simulink model "UAV_Research_Environment"  (R2025a)
settings: Solver=ode23t  StartTime=0.0  StopTime=130  MaxStep=2e-3  RelTol=1e-4  AbsTol=1e-3  EnableMultiTasking=on
InitFcn:
  | skipInitialization = false;
  | 
  | if evalin('base', ...
  |         'exist(''CONTROLLER_TUNING_ACTIVE'',''var'')')
  | 
  |     skipInitialization = evalin('base', ...
  |         'logical(CONTROLLER_TUNING_ACTIVE)');
  | end
  | 
  | if ~skipInitialization
  | 
  |     icraControllerPrepared = false;
  | 
  |     hasICRAVariables = evalin('base', ...
  |         ['exist(''AUTOPILOT'',''var'') && ' ...
  |          'exist(''ICRA_ACTIVE_CONTROLLER'',''var'') && ' ...
  |          'exist(''ICRA_ACTIVE_RUN_ID'',''var'')']);
  | 
  |     if hasICRAVariables
  | 
  |         icraControllerPrepared = evalin('base', ...
  |             ['isstruct(AUTOPILOT) && ' ...
  |              'isfield(AUTOPILOT,''info'') && ' ...
  |              'isfield(AUTOPILOT.info,''ICRAControllerID'') && ' ...
  |              'strcmp(string(AUTOPILOT.info.ICRAControllerID), ' ...
  |                     'string(ICRA_ACTIVE_CONTROLLER))']);
  | 
  |     end
  | 
  |     if icraControllerPrepared
  |         skipInitialization = true;
  |     end
  | end
  | 
  | if ~skipInitialization
  | 
  |     mdl = bdroot;
  | 
  |     mdl_file = get_param(mdl, 'FileName');
  | 
  |     project_root = fileparts(mdl_file);
  | 
  |     init_file = fullfile(project_root, 'initialize_project.m');
  | 
  |     if exist(init_file, 'file')
  | 
  |         run(init_file);
  | 
  |     else
  | 
  |         error('initialize_project.m was not found in the model folder.');
  | 
  |     end
  | end
values from neighbouring files (symbols this model uses):
  A_UAV = struct()    [UAV_analytical.m]
  AUTOPILOT = struct()    [UAV_autopilot.m]
  B_UAV = struct()    [UAV_block.m]
  D = A_UAV.source.propeller_diameter_m    [UAV_analytical.m]    (also in plot_controller_results.m = permute(                  D,                  order); plot_estimator_results.m = permute(              D,              order); plot_mission_results.m = permute(                  D,                  order); plot_touchdown_diagnostics.m = permute(                  D,                  order))
  OPERATOR_MODE = OPERATOR_MODE_MANUAL    [initialize_project.m]    (also in uav_remote_gui.m = uint8(0))
  P_ENV = struct()    [Environment.m]
  P_UAV = struct()    [UAV_simscape.m]
  s = sin(angle)    [uav_remote_gui.m]
  SENSOR = struct()    [UAV_sensors.m]
  TRAJECTORY_CONFIG = struct()    [UAV_trajectories.m]
  TRAJECTORY_ID = uint8(          trajectoryIDNumeric)    [UAV_trajectories.m]
  X = reshape(                  D,                  nt,                  [])    [plot_controller_results.m]    (also in plot_estimator_results.m = reshape(              D,              nt,              []); plot_mission_results.m; plot_touchdown_diagnostics.m; plot_trajectory_3d.m)
  Y = absolutePlanNED(1,:)    [plot_trajectory_3d.m]    (also in uav_remote_gui.m = positionNED(:,1))
  Z = landedCGDown -          absolutePlanNED(3,:)    [plot_trajectory_3d.m]    (also in uav_remote_gui.m = landedCGDown-positionNED(:,3))
undefined symbols (not defined in the file or in its folder): Acceleration_ref, F, fractalcoef, Light, MIL, Position_ref, Velocity_ref, Yaw_ref, YawRate_ref
libraries: sm_lib x49, nesl_utility x29, fl_lib x17, slpidlib x16, simulink x14, ee_lib x5, sdl_lib x4, aerolibwind2 x3, aerolibatmos2 x2, sensorbarometerlib x1, sensorgpslib x1, mspsensorlib x1
(part 6 of 9)

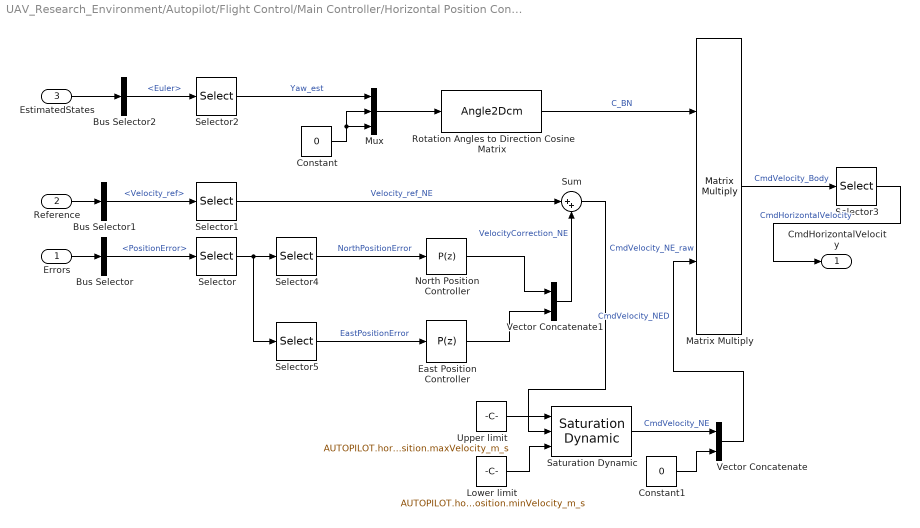
== system UAV_Research_Environment/Autopilot/Flight Control/Main Controller/Horizontal Position Control ==
  Errors : Inport
  Reference : Inport  Port=2
  EstimatedStates : Inport  Port=3
  Bus Selector : BusSelector  OutputSignals=PositionError
  Bus Selector1 : BusSelector  OutputSignals=Velocity_ref
  Bus Selector2 : BusSelector  OutputSignals=Attitude.Euler
  Constant : Constant  Value=0
  Constant1 : Constant  Value=0
  East Position Controller : slpidlib/PID Controller  Controller=P  Form=Parallel  TimeDomain=Discrete-time  UseExternalTs=off  SampleTime=AUTOPILOT.rate.controlSampleTime_s  IntegratorMethod=Forward Euler  FilterMethod=Forward Euler  ControllerParametersSource=internal  P=AUTOPILOT.horizontal.position.east.Kp  I=1  UseKiTs=off  D=0.550359987031017  UseExternalDerivativeSource=off  N=2.08014059923257  UseFilter=on  TunerSelectOption=Transfer Function Based (PID Tuner App)  InitialConditionSource=internal  InitialConditionForIntegrator=0  InitialConditionForFilter=0  DifferentiatorICPrevScaledInput=0  ExternalReset=level  TrackingMode=off  Kt=1  LimitOutput=off  SatLimitsSource=internal  UpperSaturationLimit=inf  LowerSaturationLimit=-inf  LinearizeAsGain=off  AntiWindupMode=none  Kb=1  LimitIntegrator=off  UpperIntegratorSaturationLimit=inf  LowerIntegratorSaturationLimit=-inf  POutMin=[]  POutMax=[]  IOutMin=[]  IOutMax=[]  DOutMin=[]  DOutMax=[]  NOutMin=[]  NOutMax=[]  SumOutMin=[]  SumOutMax=[]  SaturationOutMin=[]  SaturationOutMax=[]  PParamMin=[]  PParamMax=[]  IParamMin=[]  IParamMax=[]  DParamMin=[]  DParamMax=[]  NParamMin=[]  NParamMax=[]  KbParamMin=[]  KbParamMax=[]  KtParamMin=[]  KtParamMax=[]  KbOutMin=[]  KbOutMax=[]  KtOutMin=[]  KtOutMax=[]  IntegratorOutMin=[]  IntegratorOutMax=[]  FilterOutMin=[]  FilterOutMax=[]  SumI1OutMin=[]  SumI1OutMax=[]  SumI2OutMin=[]  SumI2OutMax=[]  SumI3OutMin=[]  SumI3OutMax=[]  SumI4OutMin=[]  SumI4OutMax=[]  SumDOutMin=[]  SumDOutMax=[]  DifferentiatorOutMin=[]  DifferentiatorOutMax=[]  FilterDiffOutCoefMin=[]  FilterDiffOutCoefMax=[]  ReciprocalOutMin=[]  ReciprocalOutMax=[]  SumDenOutMin=[]  SumDenOutMax=[]  SumNumOutMin=[]  SumNumOutMax=[]  DivideOutMin=[]  DivideOutMax=[]  UdiffTsProdOutMin=[]  UdiffTsProdOutMax=[]  NTsProdOutMin=[]  NTsProdOutMax=[]  UintegralTsProdOutMin=[]  UintegralTsProdOutMax=[]  UngainTsProdOutMin=[]  UngainTsProdOutMax=[]  ClampingZeroOutDataTypeStr=Inherit: Inherit via back propagation  ClampingZeroOutMin=[]  ClampingZeroOutMax=[]  FilterDenConstantOutDataTypeStr=Inherit: Inherit via back propagation  FilterDenConstantOutMin=[]  FilterDenConstantOutMax=[]  PCopyOutDataTypeStr=Inherit: Inherit via back propagation  PCopyOutMin=[]  PCopyOutMax=[]  NCopyOutDataTypeStr=Inherit: Inherit via back propagation  NCopyOutMin=[]  NCopyOutMax=[]  IntegratorContinuousStateAttributes=''  IntegratorStateMustResolveToSignalObject=off  IntegratorRTWStateStorageClass=Auto  FilterContinuousStateAttributes=''  FilterStateMustResolveToSignalObject=off  FilterRTWStateStorageClass=Auto  ParallelPVariant=InternalParameters  IdealPVariant=Disabled  IVariant=Disabled  DVariant=Disabled  IntegratorVariant=Disabled  SatVariant=Disabled  AWVariant=Disabled  PCopyVariant=Disabled  TRVariant=Disabled  FdbkBlocksVariant=Forward  IdealPFdbkVariant=Disabled  SatFdbkVariant=Disabled  DerivativeFilterVariant=Disabled  NVariant=Disabled  NCopyVariant=Disabled_SignalSpec  FilterICVariant=Disabled  IntegratorICVariant=Disabled  ExternalResetVariant=Disabled  TRSumVariant=Passthrough  SumFdbkVariant=Disabled  SumVariant=Passthrough_P  TsampFilterVariant=InternalTs  TsampNgainVariant=Passthrough  TsampIntegralVariant=Disabled_SignalSpec  ExternalSaturationOutDataTypeStr=Inherit: Same as second input  DerivativeSourceVariant=Disabled  PreIntVariant=InternalPreInt
      settings: LibrarySourceBlock=simulink/Discrete/Discrete PID Controller
  Lower limit : Constant  Value=AUTOPILOT.horizontal.position.minVelocity_m_s
  Matrix Multiply : Product  Multiplication=Matrix(*)
  Mux : Mux  Inputs=3
  North Position Controller : slpidlib/PID Controller  Controller=P  Form=Parallel  TimeDomain=Discrete-time  UseExternalTs=off  SampleTime=AUTOPILOT.rate.controlSampleTime_s  IntegratorMethod=Forward Euler  FilterMethod=Forward Euler  ControllerParametersSource=internal  P=AUTOPILOT.horizontal.position.north.Kp  I=1  UseKiTs=off  D=0  UseExternalDerivativeSource=off  N=100  UseFilter=on  TunerSelectOption=Transfer Function Based (PID Tuner App)  InitialConditionSource=internal  InitialConditionForIntegrator=0  InitialConditionForFilter=0  DifferentiatorICPrevScaledInput=0  ExternalReset=level  TrackingMode=off  Kt=1  LimitOutput=off  SatLimitsSource=internal  UpperSaturationLimit=inf  LowerSaturationLimit=-inf  LinearizeAsGain=off  AntiWindupMode=none  Kb=1  LimitIntegrator=off  UpperIntegratorSaturationLimit=inf  LowerIntegratorSaturationLimit=-inf  POutMin=[]  POutMax=[]  IOutMin=[]  IOutMax=[]  DOutMin=[]  DOutMax=[]  NOutMin=[]  NOutMax=[]  SumOutMin=[]  SumOutMax=[]  SaturationOutMin=[]  SaturationOutMax=[]  PParamMin=[]  PParamMax=[]  IParamMin=[]  IParamMax=[]  DParamMin=[]  DParamMax=[]  NParamMin=[]  NParamMax=[]  KbParamMin=[]  KbParamMax=[]  KtParamMin=[]  KtParamMax=[]  KbOutMin=[]  KbOutMax=[]  KtOutMin=[]  KtOutMax=[]  IntegratorOutMin=[]  IntegratorOutMax=[]  FilterOutMin=[]  FilterOutMax=[]  SumI1OutMin=[]  SumI1OutMax=[]  SumI2OutMin=[]  SumI2OutMax=[]  SumI3OutMin=[]  SumI3OutMax=[]  SumI4OutMin=[]  SumI4OutMax=[]  SumDOutMin=[]  SumDOutMax=[]  DifferentiatorOutMin=[]  DifferentiatorOutMax=[]  FilterDiffOutCoefMin=[]  FilterDiffOutCoefMax=[]  ReciprocalOutMin=[]  ReciprocalOutMax=[]  SumDenOutMin=[]  SumDenOutMax=[]  SumNumOutMin=[]  SumNumOutMax=[]  DivideOutMin=[]  DivideOutMax=[]  UdiffTsProdOutMin=[]  UdiffTsProdOutMax=[]  NTsProdOutMin=[]  NTsProdOutMax=[]  UintegralTsProdOutMin=[]  UintegralTsProdOutMax=[]  UngainTsProdOutMin=[]  UngainTsProdOutMax=[]  ClampingZeroOutDataTypeStr=Inherit: Inherit via back propagation  ClampingZeroOutMin=[]  ClampingZeroOutMax=[]  FilterDenConstantOutDataTypeStr=Inherit: Inherit via back propagation  FilterDenConstantOutMin=[]  FilterDenConstantOutMax=[]  PCopyOutDataTypeStr=Inherit: Inherit via back propagation  PCopyOutMin=[]  PCopyOutMax=[]  NCopyOutDataTypeStr=Inherit: Inherit via back propagation  NCopyOutMin=[]  NCopyOutMax=[]  IntegratorContinuousStateAttributes=''  IntegratorStateMustResolveToSignalObject=off  IntegratorRTWStateStorageClass=Auto  FilterContinuousStateAttributes=''  FilterStateMustResolveToSignalObject=off  FilterRTWStateStorageClass=Auto  ParallelPVariant=InternalParameters  IdealPVariant=Disabled  IVariant=Disabled  DVariant=Disabled  IntegratorVariant=Disabled  SatVariant=Disabled  AWVariant=Disabled  PCopyVariant=Disabled  TRVariant=Disabled  FdbkBlocksVariant=Forward  IdealPFdbkVariant=Disabled  SatFdbkVariant=Disabled  DerivativeFilterVariant=Disabled  NVariant=Disabled  NCopyVariant=Disabled_SignalSpec  FilterICVariant=Disabled  IntegratorICVariant=Disabled  ExternalResetVariant=Disabled  TRSumVariant=Passthrough  SumFdbkVariant=Disabled  SumVariant=Passthrough_P  TsampFilterVariant=InternalTs  TsampNgainVariant=Passthrough  TsampIntegralVariant=Disabled_SignalSpec  ExternalSaturationOutDataTypeStr=Inherit: Same as second input  DerivativeSourceVariant=Disabled  PreIntVariant=InternalPreInt
      settings: LibrarySourceBlock=simulink/Discrete/Discrete PID Controller
  Rotation Angles to Direction Cosine Matrix : Angle2Dcm
      settings: AttributesFormatString=Rotation Order: %<rotationOrder>
  Saturation Dynamic : simulink/Discontinuities/Saturation Dynamic  OutMin=[]  OutMax=[]  OutDataTypeStr=Inherit: Same as second input  OutDataType=fixdt(1, 16)  OutScaling=2^-10  DoSatur=off
  Selector : Selector  InputPortWidth=3  IndexOptions=Index vector (dialog)  Indices=[1 2]  OutputSizes=1
  Selector1 : Selector  InputPortWidth=3  IndexOptions=Index vector (dialog)  Indices=[1 2]  OutputSizes=1
  Selector2 : Selector  InputPortWidth=3  IndexOptions=Index vector (dialog)  Indices=3  OutputSizes=1
  Selector3 : Selector  InputPortWidth=3  IndexOptions=Index vector (dialog)  Indices=[1 2]  OutputSizes=1
  Selector4 : Selector  InputPortWidth=2  IndexOptions=Index vector (dialog)  Indices=1  OutputSizes=1
  Selector5 : Selector  InputPortWidth=2  IndexOptions=Index vector (dialog)  Indices=2  OutputSizes=1
  Sum : Sum  Inputs=|++
  Upper limit : Constant  Value=AUTOPILOT.horizontal.position.maxVelocity_m_s
  Vector Concatenate : Concatenate
  Vector Concatenate1 : Concatenate
  CmdHorizontalVelocity : Outport
  wires:
  Errors/1 -> Bus Selector/1
  Bus Selector/1 -> Selector/1  "<PositionError>"
  Reference/1 -> Bus Selector1/1
  Bus Selector1/1 -> Selector1/1  "<Velocity_ref>"
  EstimatedStates/1 -> Bus Selector2/1
  Bus Selector2/1 -> Selector2/1  "<Euler>"
  Selector/1 -> Selector5/1, Selector4/1
  Vector Concatenate1/1 -> Sum/2  "VelocityCorrection_NE"
  Selector1/1 -> Sum/1  "Velocity_ref_NE"
  Sum/1 -> Saturation Dynamic/2  "CmdVelocity_NE_raw"
  Saturation Dynamic/1 -> Vector Concatenate/1  "CmdVelocity_NE"
  Upper limit/1 -> Saturation Dynamic/1
  Lower limit/1 -> Saturation Dynamic/3
  Selector2/1 -> Mux/1  "Yaw_est"
  Constant/1 -> Mux/2, Mux/3
  Mux/1 -> Rotation Angles to Direction Cosine Matrix/1
  Rotation Angles to Direction Cosine Matrix/1 -> Matrix Multiply/1  "C_BN"
  Constant1/1 -> Vector Concatenate/2
  Vector Concatenate/1 -> Matrix Multiply/2  "CmdVelocity_NED"
  Matrix Multiply/1 -> Selector3/1  "CmdVelocity_Body"
  Selector3/1 -> CmdHorizontalVelocity/1  "CmdHorizontalVelocity"
  Selector4/1 -> North Position Controller/1  "NorthPositionError"
  Selector5/1 -> East Position Controller/1  "EastPositionError"
  North Position Controller/1 -> Vector Concatenate1/1
  East Position Controller/1 -> Vector Concatenate1/2

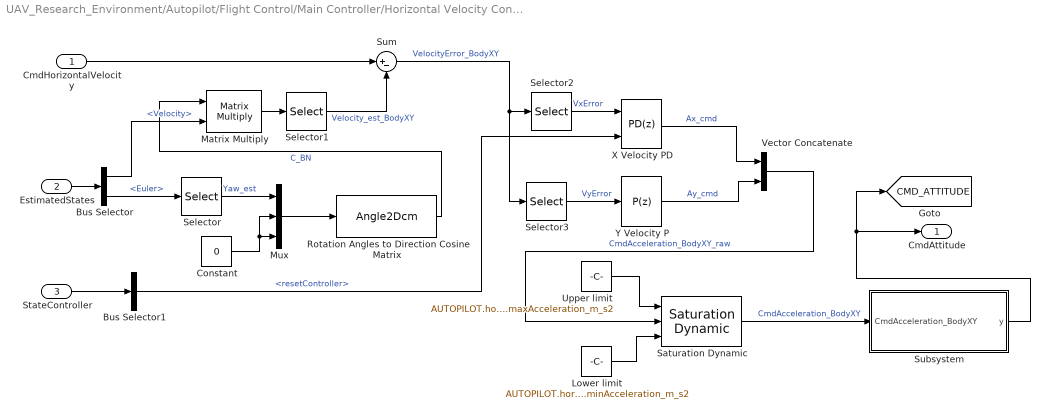
== system UAV_Research_Environment/Autopilot/Flight Control/Main Controller/Horizontal Velocity Control ==
  CmdHorizontalVelocity : Inport
  EstimatedStates : Inport  Port=2
  StateController : Inport  Port=3
  Bus Selector : BusSelector  OutputSignals=Velocity,Attitude.Euler
  Bus Selector1 : BusSelector  OutputSignals=resetController
  Constant : Constant  Value=0
  Lower limit : Constant  Value=AUTOPILOT.horizontal.velocity.minAcceleration_m_s2
  Matrix Multiply : Product  Multiplication=Matrix(*)
  Mux : Mux  Inputs=3
  Rotation Angles to Direction Cosine Matrix : Angle2Dcm
      settings: AttributesFormatString=Rotation Order: %<rotationOrder>
  Saturation Dynamic : simulink/Discontinuities/Saturation Dynamic  OutMin=[]  OutMax=[]  OutDataTypeStr=Inherit: Same as second input  OutDataType=fixdt(1, 16)  OutScaling=2^-10  DoSatur=off
  Selector : Selector  InputPortWidth=3  IndexOptions=Index vector (dialog)  Indices=3  OutputSizes=1
  Selector1 : Selector  InputPortWidth=3  IndexOptions=Index vector (dialog)  Indices=[1 2]  OutputSizes=1
  Selector2 : Selector  InputPortWidth=2  IndexOptions=Index vector (dialog)  Indices=1  OutputSizes=1
  Selector3 : Selector  InputPortWidth=2  IndexOptions=Index vector (dialog)  Indices=2  OutputSizes=1
  Subsystem : Subsystem
  Sum : Sum  Inputs=|+-
  Upper limit : Constant  Value=AUTOPILOT.horizontal.velocity.maxAcceleration_m_s2
  Vector Concatenate : Concatenate
  X Velocity PD : slpidlib/PID Controller  Controller=PD  Form=Parallel  TimeDomain=Discrete-time  UseExternalTs=off  SampleTime=AUTOPILOT.rate.controlSampleTime_s  IntegratorMethod=Forward Euler  FilterMethod=Forward Euler  ControllerParametersSource=internal  P=AUTOPILOT.horizontal.velocity.x.Kp  I=AUTOPILOT.horizontal.velocity.Ki  UseKiTs=off  D=AUTOPILOT.horizontal.velocity.x.Kd  UseExternalDerivativeSource=off  N=AUTOPILOT.horizontal.velocity.x.N  UseFilter=on  TunerSelectOption=Transfer Function Based (PID Tuner App)  InitialConditionSource=internal  InitialConditionForIntegrator=0  InitialConditionForFilter=0  DifferentiatorICPrevScaledInput=0  ExternalReset=level  TrackingMode=off  Kt=1  LimitOutput=off  SatLimitsSource=internal  UpperSaturationLimit=inf  LowerSaturationLimit=-inf  LinearizeAsGain=off  AntiWindupMode=none  Kb=1  LimitIntegrator=off  UpperIntegratorSaturationLimit=inf  LowerIntegratorSaturationLimit=-inf  POutMin=[]  POutMax=[]  IOutMin=[]  IOutMax=[]  DOutMin=[]  DOutMax=[]  NOutMin=[]  NOutMax=[]  SumOutMin=[]  SumOutMax=[]  SaturationOutMin=[]  SaturationOutMax=[]  PParamMin=[]  PParamMax=[]  IParamMin=[]  IParamMax=[]  DParamMin=[]  DParamMax=[]  NParamMin=[]  NParamMax=[]  KbParamMin=[]  KbParamMax=[]  KtParamMin=[]  KtParamMax=[]  KbOutMin=[]  KbOutMax=[]  KtOutMin=[]  KtOutMax=[]  IntegratorOutMin=[]  IntegratorOutMax=[]  FilterOutMin=[]  FilterOutMax=[]  SumI1OutMin=[]  SumI1OutMax=[]  SumI2OutMin=[]  SumI2OutMax=[]  SumI3OutMin=[]  SumI3OutMax=[]  SumI4OutMin=[]  SumI4OutMax=[]  SumDOutMin=[]  SumDOutMax=[]  DifferentiatorOutMin=[]  DifferentiatorOutMax=[]  FilterDiffOutCoefMin=[]  FilterDiffOutCoefMax=[]  ReciprocalOutMin=[]  ReciprocalOutMax=[]  SumDenOutMin=[]  SumDenOutMax=[]  SumNumOutMin=[]  SumNumOutMax=[]  DivideOutMin=[]  DivideOutMax=[]  UdiffTsProdOutMin=[]  UdiffTsProdOutMax=[]  NTsProdOutMin=[]  NTsProdOutMax=[]  UintegralTsProdOutMin=[]  UintegralTsProdOutMax=[]  UngainTsProdOutMin=[]  UngainTsProdOutMax=[]  ClampingZeroOutDataTypeStr=Inherit: Inherit via back propagation  ClampingZeroOutMin=[]  ClampingZeroOutMax=[]  FilterDenConstantOutDataTypeStr=Inherit: Inherit via back propagation  FilterDenConstantOutMin=[]  FilterDenConstantOutMax=[]  PCopyOutDataTypeStr=Inherit: Inherit via back propagation  PCopyOutMin=[]  PCopyOutMax=[]  NCopyOutDataTypeStr=Inherit: Inherit via back propagation  NCopyOutMin=[]  NCopyOutMax=[]  IntegratorContinuousStateAttributes=''  IntegratorStateMustResolveToSignalObject=off  IntegratorRTWStateStorageClass=Auto  FilterContinuousStateAttributes=''  FilterStateMustResolveToSignalObject=off  FilterRTWStateStorageClass=Auto  ParallelPVariant=InternalParameters  IdealPVariant=Disabled  IVariant=Disabled  DVariant=InternalParameters  IntegratorVariant=Disabled  SatVariant=Disabled  AWVariant=Disabled  PCopyVariant=Disabled  TRVariant=Disabled  FdbkBlocksVariant=Forward  IdealPFdbkVariant=Disabled  SatFdbkVariant=Disabled  DerivativeFilterVariant=ForwardEulerFilter  NVariant=InternalParameters  NCopyVariant=Disabled  FilterICVariant=InternalICsFilter  IntegratorICVariant=Disabled  ExternalResetVariant=ExternalReset  TRSumVariant=Passthrough  SumFdbkVariant=Disabled  SumVariant=Sum_PD  TsampFilterVariant=InternalTs  TsampNgainVariant=Passthrough  TsampIntegralVariant=Disabled_SignalSpec  ExternalSaturationOutDataTypeStr=Inherit: Same as second input  DerivativeSourceVariant=ErrorSignal  PreIntVariant=InternalPreInt
      settings: LibrarySourceBlock=simulink/Discrete/Discrete PID Controller
  Y Velocity P : slpidlib/PID Controller  Controller=P  Form=Parallel  TimeDomain=Discrete-time  UseExternalTs=off  SampleTime=AUTOPILOT.rate.controlSampleTime_s  IntegratorMethod=Forward Euler  FilterMethod=Forward Euler  ControllerParametersSource=internal  P=AUTOPILOT.horizontal.velocity.y.Kp  I=AUTOPILOT.horizontal.velocity.Ki  UseKiTs=off  D=AUTOPILOT.horizontal.velocity.Kd  UseExternalDerivativeSource=off  N=AUTOPILOT.horizontal.velocity.N  UseFilter=on  TunerSelectOption=Transfer Function Based (PID Tuner App)  InitialConditionSource=internal  InitialConditionForIntegrator=0  InitialConditionForFilter=0  DifferentiatorICPrevScaledInput=0  ExternalReset=level  TrackingMode=off  Kt=1  LimitOutput=off  SatLimitsSource=internal  UpperSaturationLimit=inf  LowerSaturationLimit=-inf  LinearizeAsGain=off  AntiWindupMode=none  Kb=1  LimitIntegrator=off  UpperIntegratorSaturationLimit=inf  LowerIntegratorSaturationLimit=-inf  POutMin=[]  POutMax=[]  IOutMin=[]  IOutMax=[]  DOutMin=[]  DOutMax=[]  NOutMin=[]  NOutMax=[]  SumOutMin=[]  SumOutMax=[]  SaturationOutMin=[]  SaturationOutMax=[]  PParamMin=[]  PParamMax=[]  IParamMin=[]  IParamMax=[]  DParamMin=[]  DParamMax=[]  NParamMin=[]  NParamMax=[]  KbParamMin=[]  KbParamMax=[]  KtParamMin=[]  KtParamMax=[]  KbOutMin=[]  KbOutMax=[]  KtOutMin=[]  KtOutMax=[]  IntegratorOutMin=[]  IntegratorOutMax=[]  FilterOutMin=[]  FilterOutMax=[]  SumI1OutMin=[]  SumI1OutMax=[]  SumI2OutMin=[]  SumI2OutMax=[]  SumI3OutMin=[]  SumI3OutMax=[]  SumI4OutMin=[]  SumI4OutMax=[]  SumDOutMin=[]  SumDOutMax=[]  DifferentiatorOutMin=[]  DifferentiatorOutMax=[]  FilterDiffOutCoefMin=[]  FilterDiffOutCoefMax=[]  ReciprocalOutMin=[]  ReciprocalOutMax=[]  SumDenOutMin=[]  SumDenOutMax=[]  SumNumOutMin=[]  SumNumOutMax=[]  DivideOutMin=[]  DivideOutMax=[]  UdiffTsProdOutMin=[]  UdiffTsProdOutMax=[]  NTsProdOutMin=[]  NTsProdOutMax=[]  UintegralTsProdOutMin=[]  UintegralTsProdOutMax=[]  UngainTsProdOutMin=[]  UngainTsProdOutMax=[]  ClampingZeroOutDataTypeStr=Inherit: Inherit via back propagation  ClampingZeroOutMin=[]  ClampingZeroOutMax=[]  FilterDenConstantOutDataTypeStr=Inherit: Inherit via back propagation  FilterDenConstantOutMin=[]  FilterDenConstantOutMax=[]  PCopyOutDataTypeStr=Inherit: Inherit via back propagation  PCopyOutMin=[]  PCopyOutMax=[]  NCopyOutDataTypeStr=Inherit: Inherit via back propagation  NCopyOutMin=[]  NCopyOutMax=[]  IntegratorContinuousStateAttributes=''  IntegratorStateMustResolveToSignalObject=off  IntegratorRTWStateStorageClass=Auto  FilterContinuousStateAttributes=''  FilterStateMustResolveToSignalObject=off  FilterRTWStateStorageClass=Auto  ParallelPVariant=InternalParameters  IdealPVariant=Disabled  IVariant=Disabled  DVariant=Disabled  IntegratorVariant=Disabled  SatVariant=Disabled  AWVariant=Disabled  PCopyVariant=Disabled  TRVariant=Disabled  FdbkBlocksVariant=Forward  IdealPFdbkVariant=Disabled  SatFdbkVariant=Disabled  DerivativeFilterVariant=Disabled  NVariant=Disabled  NCopyVariant=Disabled_SignalSpec  FilterICVariant=Disabled  IntegratorICVariant=Disabled  ExternalResetVariant=Disabled  TRSumVariant=Passthrough  SumFdbkVariant=Disabled  SumVariant=Passthrough_P  TsampFilterVariant=InternalTs  TsampNgainVariant=Passthrough  TsampIntegralVariant=Disabled_SignalSpec  ExternalSaturationOutDataTypeStr=Inherit: Same as second input  DerivativeSourceVariant=Disabled  PreIntVariant=InternalPreInt
      settings: LibrarySourceBlock=simulink/Discrete/Discrete PID Controller
  CmdAttitude : Outport
  tag scope: CMD_ATTITUDE=global
  wires:
  EstimatedStates/1 -> Bus Selector/1
  StateController/1 -> Bus Selector1/1
  Bus Selector/2 -> Selector/1  "<Euler>"
  Selector/1 -> Mux/1  "Yaw_est"
  Constant/1 -> Mux/2, Mux/3
  Mux/1 -> Rotation Angles to Direction Cosine Matrix/1
  Rotation Angles to Direction Cosine Matrix/1 -> Matrix Multiply/1  "C_BN"
  Bus Selector/1 -> Matrix Multiply/2  "<Velocity>"
  Matrix Multiply/1 -> Selector1/1
  Selector1/1 -> Sum/2  "Velocity_est_BodyXY"
  CmdHorizontalVelocity/1 -> Sum/1
  Sum/1 -> Selector3/1, Selector2/1  "VelocityError_BodyXY"
  Bus Selector1/1 -> X Velocity PD/2  "<resetController>"
  Vector Concatenate/1 -> Saturation Dynamic/2  "CmdAcceleration_BodyXY_raw"
  Upper limit/1 -> Saturation Dynamic/1
  Lower limit/1 -> Saturation Dynamic/3
  Saturation Dynamic/1 -> Subsystem/1(CmdAcceleration_BodyXY)  "CmdAcceleration_BodyXY"
  Selector2/1 -> X Velocity PD/1  "VxError"
  Selector3/1 -> Y Velocity P/1  "VyError"
  Y Velocity P/1 -> Vector Concatenate/2  "Ay_cmd"
  Subsystem/1(y) -> [CMD_ATTITUDE], CmdAttitude/1
  X Velocity PD/1 -> Vector Concatenate/1  "Ax_cmd"

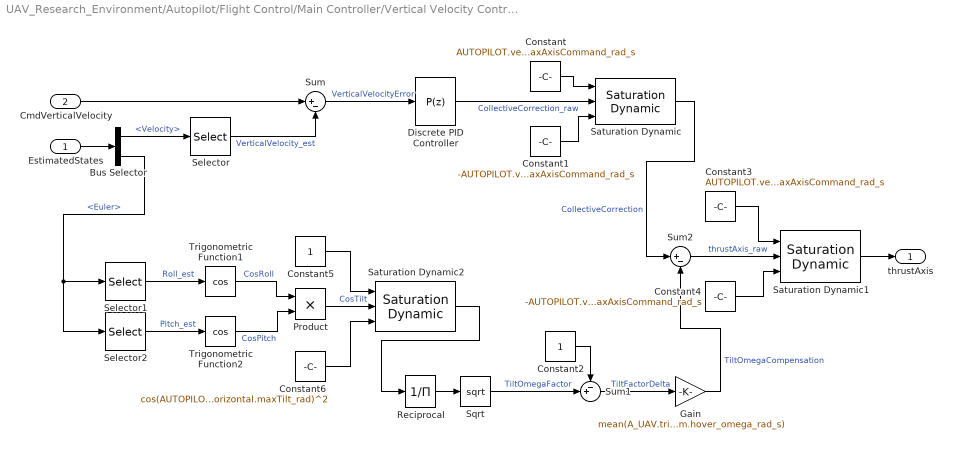
== system UAV_Research_Environment/Autopilot/Flight Control/Main Controller/Vertical Velocity Control ==
  EstimatedStates : Inport
  CmdVerticalVelocity : Inport  Port=2
  Bus Selector : BusSelector  OutputSignals=Velocity,Attitude.Euler
  Constant : Constant  Value=AUTOPILOT.vertical.velocity.maxAxisCommand_rad_s
  Constant1 : Constant  Value=-AUTOPILOT.vertical.velocity.maxAxisCommand_rad_s
  Constant2 : Constant
  Constant3 : Constant  Value=AUTOPILOT.vertical.velocity.maxAxisCommand_rad_s
  Constant4 : Constant  Value=-AUTOPILOT.vertical.velocity.maxAxisCommand_rad_s
  Constant5 : Constant
  Constant6 : Constant  Value=cos(AUTOPILOT.horizontal.maxTilt_rad)^2
  Discrete PID Controller : slpidlib/PID Controller  Controller=P  Form=Parallel  TimeDomain=Discrete-time  UseExternalTs=off  SampleTime=AUTOPILOT.rate.controlSampleTime_s  IntegratorMethod=Forward Euler  FilterMethod=Forward Euler  ControllerParametersSource=internal  P=AUTOPILOT.vertical.velocity.Kp  I=AUTOPILOT.vertical.velocity.Ki  UseKiTs=off  D=AUTOPILOT.vertical.velocity.Kd  UseExternalDerivativeSource=off  N=AUTOPILOT.vertical.velocity.N  UseFilter=on  TunerSelectOption=Transfer Function Based (PID Tuner App)  InitialConditionSource=internal  InitialConditionForIntegrator=0  InitialConditionForFilter=0  DifferentiatorICPrevScaledInput=0  ExternalReset=level  TrackingMode=off  Kt=1  LimitOutput=off  SatLimitsSource=internal  UpperSaturationLimit=inf  LowerSaturationLimit=-inf  LinearizeAsGain=off  AntiWindupMode=clamping  Kb=1  LimitIntegrator=on  UpperIntegratorSaturationLimit=AUTOPILOT.vertical.velocity.integratorUpperLimit  LowerIntegratorSaturationLimit=AUTOPILOT.vertical.velocity.integratorLowerLimit  POutMin=[]  POutMax=[]  IOutMin=[]  IOutMax=[]  DOutMin=[]  DOutMax=[]  NOutMin=[]  NOutMax=[]  SumOutMin=[]  SumOutMax=[]  SaturationOutMin=[]  SaturationOutMax=[]  PParamMin=[]  PParamMax=[]  IParamMin=[]  IParamMax=[]  DParamMin=[]  DParamMax=[]  NParamMin=[]  NParamMax=[]  KbParamMin=[]  KbParamMax=[]  KtParamMin=[]  KtParamMax=[]  KbOutMin=[]  KbOutMax=[]  KtOutMin=[]  KtOutMax=[]  IntegratorOutMin=[]  IntegratorOutMax=[]  FilterOutMin=[]  FilterOutMax=[]  SumI1OutMin=[]  SumI1OutMax=[]  SumI2OutMin=[]  SumI2OutMax=[]  SumI3OutMin=[]  SumI3OutMax=[]  SumI4OutMin=[]  SumI4OutMax=[]  SumDOutMin=[]  SumDOutMax=[]  DifferentiatorOutMin=[]  DifferentiatorOutMax=[]  FilterDiffOutCoefMin=[]  FilterDiffOutCoefMax=[]  ReciprocalOutMin=[]  ReciprocalOutMax=[]  SumDenOutMin=[]  SumDenOutMax=[]  SumNumOutMin=[]  SumNumOutMax=[]  DivideOutMin=[]  DivideOutMax=[]  UdiffTsProdOutMin=[]  UdiffTsProdOutMax=[]  NTsProdOutMin=[]  NTsProdOutMax=[]  UintegralTsProdOutMin=[]  UintegralTsProdOutMax=[]  UngainTsProdOutMin=[]  UngainTsProdOutMax=[]  ClampingZeroOutDataTypeStr=Inherit: Inherit via back propagation  ClampingZeroOutMin=[]  ClampingZeroOutMax=[]  FilterDenConstantOutDataTypeStr=Inherit: Inherit via back propagation  FilterDenConstantOutMin=[]  FilterDenConstantOutMax=[]  PCopyOutDataTypeStr=Inherit: Inherit via back propagation  PCopyOutMin=[]  PCopyOutMax=[]  NCopyOutDataTypeStr=Inherit: Inherit via back propagation  NCopyOutMin=[]  NCopyOutMax=[]  IntegratorContinuousStateAttributes=''  IntegratorStateMustResolveToSignalObject=off  IntegratorRTWStateStorageClass=Auto  FilterContinuousStateAttributes=''  FilterStateMustResolveToSignalObject=off  FilterRTWStateStorageClass=Auto  ParallelPVariant=InternalParameters  IdealPVariant=Disabled  IVariant=Disabled  DVariant=Disabled  IntegratorVariant=Disabled  SatVariant=Disabled  AWVariant=Disabled  PCopyVariant=Disabled  TRVariant=Disabled  FdbkBlocksVariant=Forward  IdealPFdbkVariant=Disabled  SatFdbkVariant=Disabled  DerivativeFilterVariant=Disabled  NVariant=Disabled  NCopyVariant=Disabled_SignalSpec  FilterICVariant=Disabled  IntegratorICVariant=Disabled  ExternalResetVariant=Disabled  TRSumVariant=Passthrough  SumFdbkVariant=Disabled  SumVariant=Passthrough_P  TsampFilterVariant=InternalTs  TsampNgainVariant=Passthrough  TsampIntegralVariant=Disabled_SignalSpec  ExternalSaturationOutDataTypeStr=Inherit: Same as second input  DerivativeSourceVariant=Disabled  PreIntVariant=InternalPreInt
      settings: LibrarySourceBlock=simulink/Discrete/Discrete PID Controller
  Gain : Gain  Gain=mean(A_UAV.trim.hover_omega_rad_s)
  Product : Product
  Reciprocal : Product  Inputs=/
  Saturation Dynamic : simulink/Discontinuities/Saturation Dynamic  OutMin=[]  OutMax=[]  OutDataTypeStr=Inherit: Same as second input  OutDataType=fixdt(1, 16)  OutScaling=2^-10  DoSatur=off
  Saturation Dynamic1 : simulink/Discontinuities/Saturation Dynamic  OutMin=[]  OutMax=[]  OutDataTypeStr=Inherit: Same as second input  OutDataType=fixdt(1, 16)  OutScaling=2^-10  DoSatur=off
  Saturation Dynamic2 : simulink/Discontinuities/Saturation Dynamic  OutMin=[]  OutMax=[]  OutDataTypeStr=Inherit: Same as second input  OutDataType=fixdt(1, 16)  OutScaling=2^-10  DoSatur=off
  Selector : Selector  InputPortWidth=3  IndexOptions=Index vector (dialog)  Indices=3  OutputSizes=1
  Selector1 : Selector  InputPortWidth=3  IndexOptions=Index vector (dialog)  Indices=1  OutputSizes=1
  Selector2 : Selector  InputPortWidth=3  IndexOptions=Index vector (dialog)  Indices=2  OutputSizes=1
  Sqrt : Sqrt
  Sum : Sum  Inputs=|+-
  Sum1 : Sum  Inputs=-+|
  Sum2 : Sum  Inputs=|+-
  Trigonometric Function1 : Trigonometry  Operator=cos
  Trigonometric Function2 : Trigonometry  Operator=cos
  thrustAxis : Outport
  wires:
  EstimatedStates/1 -> Bus Selector/1
  Bus Selector/1 -> Selector/1  "<Velocity>"
  Selector/1 -> Sum/2  "VerticalVelocity_est"
  CmdVerticalVelocity/1 -> Sum/1
  Sum/1 -> Discrete PID Controller/1  "VerticalVelocityError"
  Discrete PID Controller/1 -> Saturation Dynamic/2  "CollectiveCorrection_raw"
  Constant/1 -> Saturation Dynamic/1
  Constant1/1 -> Saturation Dynamic/3
  Saturation Dynamic/1 -> Sum2/1  "CollectiveCorrection"
  Selector1/1 -> Trigonometric Function1/1  "Roll_est"
  Selector2/1 -> Trigonometric Function2/1  "Pitch_est"
  Trigonometric Function1/1 -> Product/1  "CosRoll"
  Trigonometric Function2/1 -> Product/2  "CosPitch"
  Reciprocal/1 -> Sqrt/1
  Bus Selector/2 -> Selector2/1, Selector1/1  "<Euler>"
  Sum1/1 -> Gain/1  "TiltFactorDelta"
  Gain/1 -> Sum2/2  "TiltOmegaCompensation"
  Sum2/1 -> Saturation Dynamic1/2  "thrustAxis_raw"
  Saturation Dynamic1/1 -> thrustAxis/1
  Constant3/1 -> Saturation Dynamic1/1
  Constant4/1 -> Saturation Dynamic1/3
  Product/1 -> Saturation Dynamic2/2  "CosTilt"
  Saturation Dynamic2/1 -> Reciprocal/1
  Constant5/1 -> Saturation Dynamic2/1
  Constant6/1 -> Saturation Dynamic2/3
  Sqrt/1 -> Sum1/2  "TiltOmegaFactor"
  Constant2/1 -> Sum1/1

== system UAV_Research_Environment/Autopilot/Flight Control/Main Controller/Yaw Angle Control ==
  Errors : Inport
  Reference : Inport  Port=2
  Bus Selector : BusSelector  OutputSignals=YawError
  Bus Selector1 : BusSelector  OutputSignals=YawRate_ref
  Constant : Constant  Value=AUTOPILOT.yaw.angle.maxYawRate_rad_s
  Constant1 : Constant  Value=AUTOPILOT.yaw.angle.minYawRate_rad_s
  Discrete PID Controller : slpidlib/PID Controller  Controller=P  Form=Parallel  TimeDomain=Discrete-time  UseExternalTs=off  SampleTime=AUTOPILOT.rate.controlSampleTime_s  IntegratorMethod=Forward Euler  FilterMethod=Forward Euler  ControllerParametersSource=internal  P=AUTOPILOT.yaw.angle.Kp  I=AUTOPILOT.yaw.angle.Ki  UseKiTs=off  D=AUTOPILOT.yaw.angle.Kd  UseExternalDerivativeSource=off  N=AUTOPILOT.yaw.angle.N  UseFilter=on  TunerSelectOption=Transfer Function Based (PID Tuner App)  InitialConditionSource=internal  InitialConditionForIntegrator=0  InitialConditionForFilter=0  DifferentiatorICPrevScaledInput=0  ExternalReset=level  TrackingMode=off  Kt=1  LimitOutput=off  SatLimitsSource=internal  UpperSaturationLimit=inf  LowerSaturationLimit=-inf  LinearizeAsGain=off  AntiWindupMode=none  Kb=1  LimitIntegrator=off  UpperIntegratorSaturationLimit=inf  LowerIntegratorSaturationLimit=-inf  POutMin=[]  POutMax=[]  IOutMin=[]  IOutMax=[]  DOutMin=[]  DOutMax=[]  NOutMin=[]  NOutMax=[]  SumOutMin=[]  SumOutMax=[]  SaturationOutMin=[]  SaturationOutMax=[]  PParamMin=[]  PParamMax=[]  IParamMin=[]  IParamMax=[]  DParamMin=[]  DParamMax=[]  NParamMin=[]  NParamMax=[]  KbParamMin=[]  KbParamMax=[]  KtParamMin=[]  KtParamMax=[]  KbOutMin=[]  KbOutMax=[]  KtOutMin=[]  KtOutMax=[]  IntegratorOutMin=[]  IntegratorOutMax=[]  FilterOutMin=[]  FilterOutMax=[]  SumI1OutMin=[]  SumI1OutMax=[]  SumI2OutMin=[]  SumI2OutMax=[]  SumI3OutMin=[]  SumI3OutMax=[]  SumI4OutMin=[]  SumI4OutMax=[]  SumDOutMin=[]  SumDOutMax=[]  DifferentiatorOutMin=[]  DifferentiatorOutMax=[]  FilterDiffOutCoefMin=[]  FilterDiffOutCoefMax=[]  ReciprocalOutMin=[]  ReciprocalOutMax=[]  SumDenOutMin=[]  SumDenOutMax=[]  SumNumOutMin=[]  SumNumOutMax=[]  DivideOutMin=[]  DivideOutMax=[]  UdiffTsProdOutMin=[]  UdiffTsProdOutMax=[]  NTsProdOutMin=[]  NTsProdOutMax=[]  UintegralTsProdOutMin=[]  UintegralTsProdOutMax=[]  UngainTsProdOutMin=[]  UngainTsProdOutMax=[]  ClampingZeroOutDataTypeStr=Inherit: Inherit via back propagation  ClampingZeroOutMin=[]  ClampingZeroOutMax=[]  FilterDenConstantOutDataTypeStr=Inherit: Inherit via back propagation  FilterDenConstantOutMin=[]  FilterDenConstantOutMax=[]  PCopyOutDataTypeStr=Inherit: Inherit via back propagation  PCopyOutMin=[]  PCopyOutMax=[]  NCopyOutDataTypeStr=Inherit: Inherit via back propagation  NCopyOutMin=[]  NCopyOutMax=[]  IntegratorContinuousStateAttributes=''  IntegratorStateMustResolveToSignalObject=off  IntegratorRTWStateStorageClass=Auto  FilterContinuousStateAttributes=''  FilterStateMustResolveToSignalObject=off  FilterRTWStateStorageClass=Auto  ParallelPVariant=InternalParameters  IdealPVariant=Disabled  IVariant=Disabled  DVariant=Disabled  IntegratorVariant=Disabled  SatVariant=Disabled  AWVariant=Disabled  PCopyVariant=Disabled  TRVariant=Disabled  FdbkBlocksVariant=Forward  IdealPFdbkVariant=Disabled  SatFdbkVariant=Disabled  DerivativeFilterVariant=Disabled  NVariant=Disabled  NCopyVariant=Disabled_SignalSpec  FilterICVariant=Disabled  IntegratorICVariant=Disabled  ExternalResetVariant=Disabled  TRSumVariant=Passthrough  SumFdbkVariant=Disabled  SumVariant=Passthrough_P  TsampFilterVariant=InternalTs  TsampNgainVariant=Passthrough  TsampIntegralVariant=Disabled_SignalSpec  ExternalSaturationOutDataTypeStr=Inherit: Same as second input  DerivativeSourceVariant=Disabled  PreIntVariant=InternalPreInt
      settings: LibrarySourceBlock=simulink/Discrete/Discrete PID Controller
  Saturation Dynamic : simulink/Discontinuities/Saturation Dynamic  OutMin=[]  OutMax=[]  OutDataTypeStr=Inherit: Same as second input  OutDataType=fixdt(1, 16)  OutScaling=2^-10  DoSatur=off
  Sum : Sum  Inputs=|++
  CmdYawAngleRate : Outport
  wires:
  Errors/1 -> Bus Selector/1
  Reference/1 -> Bus Selector1/1
  Discrete PID Controller/1 -> Sum/1  "YawRateCorrection"
  Bus Selector/1 -> Discrete PID Controller/1  "<YawError>"
  Bus Selector1/1 -> Sum/2  "<YawRate_ref>"
  Sum/1 -> Saturation Dynamic/2  "CmdYawRate_raw"
  Constant1/1 -> Saturation Dynamic/3
  Constant/1 -> Saturation Dynamic/1
  Saturation Dynamic/1 -> CmdYawAngleRate/1

== system UAV_Research_Environment/UAV Plant/UAV Analytical [ODEs]/Rotational Dynamics/Gyroscopic Term ==
  "Omega_body " : Inport
  "I_Omega    " : Inport  Port=2
  Demux : Demux  Outputs=3
  Demux1 : Demux  Outputs=3
  Mux : Mux  Inputs=3
  Product{,1..5} (6 alike) : Product
  Sum : Sum  Inputs=|+-
  Sum1 : Sum  Inputs=|+-
  Sum2 : Sum  Inputs=|+-
  Gyro : Outport
  wires:
  "Omega_body "/1 -> Demux/1
  "I_Omega    "/1 -> Demux1/1
  Demux/1 -> Product4/1, Product3/1  "p"
  Demux/2 -> Product5/1, Product/1  "q"
  Demux/3 -> Product2/1, Product1/1  "r"
  Demux1/1 -> Product5/2, Product2/2  "hx"
  Demux1/2 -> Product4/2, Product1/2  "hy"
  Demux1/3 -> Product3/2, Product/2  "hz"
  Product/1 -> Sum/1
  Product1/1 -> Sum/2
  Sum/1 -> Mux/1  "Gx"
  Product2/1 -> Sum1/1
  Product3/1 -> Sum1/2
  Sum1/1 -> Mux/2  "Gy"
  Product4/1 -> Sum2/1
  Product5/1 -> Sum2/2
  Sum2/1 -> Mux/3  "Gz"
  Mux/1 -> Gyro/1

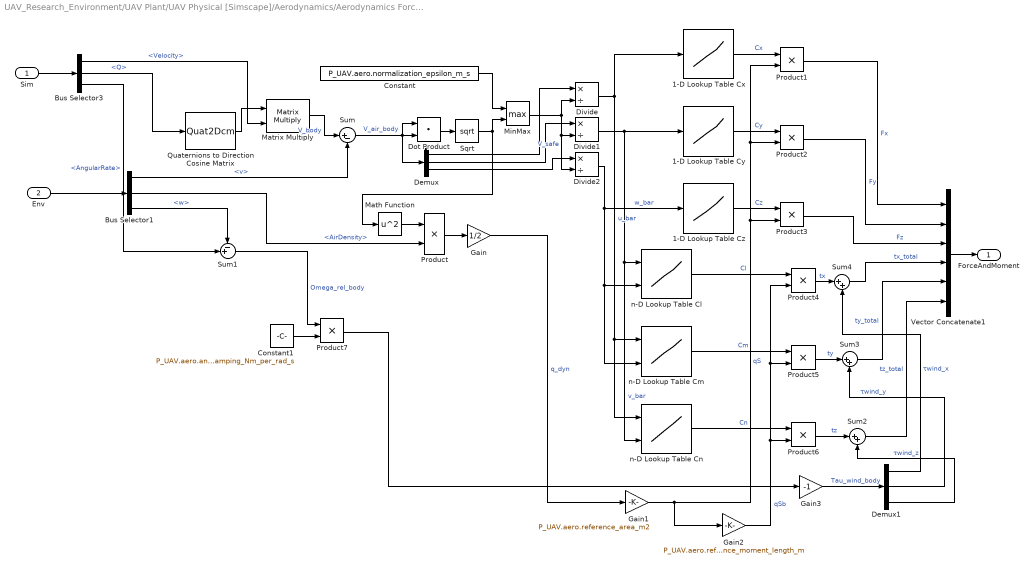
== system UAV_Research_Environment/UAV Plant/UAV Physical [Simscape]/Aerodynamics/Aerodynamics Forces and Moments ==
  Sim : Inport
  Env : Inport  Port=2
  1-D Lookup Table Cx : Lookup_n-D  NumberOfTableDimensions=1  BreakpointsForDimension1=P_UAV.aero.lookup.breakpoints  Table=P_UAV.aero.lookup.Cx  InternalRulePriority=Speed  RndMeth=Simplest
  1-D Lookup Table Cy : Lookup_n-D  NumberOfTableDimensions=1  BreakpointsForDimension1=P_UAV.aero.lookup.breakpoints  Table=P_UAV.aero.lookup.Cy  InternalRulePriority=Speed  RndMeth=Simplest
  1-D Lookup Table Cz : Lookup_n-D  NumberOfTableDimensions=1  BreakpointsForDimension1=P_UAV.aero.lookup.breakpoints  Table=P_UAV.aero.lookup.Cz  InternalRulePriority=Speed  RndMeth=Simplest
  Bus Selector1 : BusSelector  OutputSignals=Wind.v,Atmosphere.AirDensity,Wind.w
  Bus Selector3 : BusSelector  OutputSignals=Velocity,Attitude.Q,AngularRate
  Constant : Constant  Value=P_UAV.aero.normalization_epsilon_m_s
  Constant1 : Constant  Value=P_UAV.aero.angular_damping_Nm_per_rad_s
  Demux : Demux  Outputs=3
  Demux1 : Demux  Outputs=3
  Divide : Product  Inputs=*/
  Divide1 : Product  Inputs=*/
  Divide2 : Product  Inputs=*/
  Dot Product : DotProduct  OutDataTypeStr=Inherit: Inherit via internal rule
  Gain : Gain  Gain=1/2
  Gain1 : Gain  Gain=P_UAV.aero.reference_area_m2
  Gain2 : Gain  Gain=P_UAV.aero.reference_moment_length_m
  Gain3 : Gain  Gain=-1
  Math Function : Math  Operator=square
  Matrix Multiply : Product  Multiplication=Matrix(*)
  MinMax : MinMax  Function=max  Inputs=2
  Product{,1..7} (8 alike) : Product
  Quaternions to Direction Cosine Matrix : Quat2Dcm
  Sqrt : Sqrt
  Sum : Sum  Inputs=|+-
  Sum1 : Sum  Inputs=-+|
  Sum2 : Sum  Inputs=|++
  Sum3 : Sum  Inputs=|++
  Sum4 : Sum  Inputs=|++
  Vector Concatenate1 : Concatenate  NumInputs=6
  n-D Lookup Table Cl : Lookup_n-D  BreakpointsForDimension1=P_UAV.aero.lookup.breakpoints  BreakpointsForDimension2=P_UAV.aero.lookup.breakpoints  BreakpointsForDimension3=[5, 7]  Table=P_UAV.aero.lookup.Cl  InternalRulePriority=Speed  RndMeth=Simplest
      settings: InputPortMap=u0,u1
  n-D Lookup Table Cm : Lookup_n-D  BreakpointsForDimension1=P_UAV.aero.lookup.breakpoints  BreakpointsForDimension2=P_UAV.aero.lookup.breakpoints  BreakpointsForDimension3=[5, 7]  Table=P_UAV.aero.lookup.Cm  InternalRulePriority=Speed  RndMeth=Simplest
      settings: InputPortMap=u0,u1
  n-D Lookup Table Cn : Lookup_n-D  BreakpointsForDimension1=P_UAV.aero.lookup.breakpoints  BreakpointsForDimension2=P_UAV.aero.lookup.breakpoints  BreakpointsForDimension3=[5, 7]  Table=P_UAV.aero.lookup.Cn  InternalRulePriority=Speed  RndMeth=Simplest
      settings: InputPortMap=u0,u1
  ForceAndMoment : Outport
  wires:
  Sim/1 -> Bus Selector3/1
  Env/1 -> Bus Selector1/1
  Dot Product/1 -> Sqrt/1
  Quaternions to Direction Cosine Matrix/1 -> Matrix Multiply/1
  Matrix Multiply/1 -> Sum/1  "V_body"
  Bus Selector1/1 -> Sum/2  "<v>"
  Sum/1 -> Demux/1, Dot Product/1, Dot Product/2  "V_air_body"
  Constant/1 -> MinMax/1
  Sqrt/1 -> Math Function/1, MinMax/2
  Demux/1 -> Divide/1
  Demux/2 -> Divide1/1
  Demux/3 -> Divide2/1
  Divide/1 -> n-D Lookup Table Cm/1, n-D Lookup Table Cn/1, 1-D Lookup Table Cx/1  "u_bar"
  Divide1/1 -> n-D Lookup Table Cn/2, n-D Lookup Table Cl/1, 1-D Lookup Table Cy/1  "v_bar"
  Divide2/1 -> n-D Lookup Table Cl/2, n-D Lookup Table Cm/2, 1-D Lookup Table Cz/1  "w_bar"
  Bus Selector1/2 -> Product/2  "<AirDensity>"
  1-D Lookup Table Cx/1 -> Product1/1  "Cx"
  1-D Lookup Table Cy/1 -> Product2/1  "Cy"
  1-D Lookup Table Cz/1 -> Product3/1  "Cz"
  n-D Lookup Table Cl/1 -> Product4/1  "Cl"
  n-D Lookup Table Cm/1 -> Product5/1  "Cm"
  n-D Lookup Table Cn/1 -> Product6/1  "Cn"
  Math Function/1 -> Product/1
  Product/1 -> Gain/1
  Gain/1 -> Gain1/1  "q_dyn"
  Gain1/1 -> Product2/2, Product1/2, Product3/2, Gain2/1  "qS"
  Product1/1 -> Vector Concatenate1/1  "Fx"
  Product2/1 -> Vector Concatenate1/2  "Fy"
  Product3/1 -> Vector Concatenate1/3  "Fz"
  Gain2/1 -> Product6/2, Product5/2, Product4/2  "qSb"
  Vector Concatenate1/1 -> ForceAndMoment/1
  MinMax/1 -> Divide/2, Divide2/2, Divide1/2  "V_safe"
  Bus Selector1/3 -> Sum1/1  "<w>"
  Bus Selector3/3 -> Sum1/2  "<AngularRate>"
  Sum1/1 -> Product7/1  "Omega_rel_body"
  Constant1/1 -> Product7/2
  Gain3/1 -> Demux1/1  "Tau_wind_body"
  Product7/1 -> Gain3/1
  Demux1/1 -> Sum4/2  "τwind_x"
  Demux1/2 -> Sum3/2  "τwind_y"
  Demux1/3 -> Sum2/2  "τwind_z"
  Product6/1 -> Sum2/1  "tz"
  Sum2/1 -> Vector Concatenate1/6  "tz_total"
  Product5/1 -> Sum3/1  "ty"
  Sum3/1 -> Vector Concatenate1/5  "ty_total"
  Product4/1 -> Sum4/1  "tx"
  Sum4/1 -> Vector Concatenate1/4  "tx_total"
  Bus Selector3/1 -> Matrix Multiply/2  "<Velocity>"
  Bus Selector3/2 -> Quaternions to Direction Cosine Matrix/1  "<Q>"

== system UAV_Research_Environment/UAV Plant/UAV Physical [Simscape]/Motor ESC 1/Speed PI Control ==
  wCmd : Inport
  w : Inport  Port=2
  PI Controller : slpidlib/PID Controller  Controller=PI  Form=Parallel  TimeDomain=Continuous-time  UseExternalTs=off  SampleTime=-1  IntegratorMethod=Forward Euler  FilterMethod=Forward Euler  ControllerParametersSource=internal  P=P_UAV.drive.speed_pi.Kp  I=P_UAV.drive.speed_pi.Ki  UseKiTs=off  D=0.000001  UseExternalDerivativeSource=off  N=10000  UseFilter=on  TunerSelectOption=Transfer Function Based (PID Tuner App)  InitialConditionSource=internal  InitialConditionForIntegrator=0  InitialConditionForFilter=0  DifferentiatorICPrevScaledInput=0  ExternalReset=none  TrackingMode=off  Kt=1  LimitOutput=on  SatLimitsSource=internal  UpperSaturationLimit=P_UAV.drive.speed_pi.torque_limit_Nm  LowerSaturationLimit=-P_UAV.drive.speed_pi.torque_limit_Nm  LinearizeAsGain=on  AntiWindupMode=clamping  Kb=1  LimitIntegrator=off  UpperIntegratorSaturationLimit=inf  LowerIntegratorSaturationLimit=-inf  POutMin=[]  POutMax=[]  IOutMin=[]  IOutMax=[]  DOutMin=[]  DOutMax=[]  NOutMin=[]  NOutMax=[]  SumOutMin=[]  SumOutMax=[]  SaturationOutMin=[]  SaturationOutMax=[]  PParamMin=[]  PParamMax=[]  IParamMin=[]  IParamMax=[]  DParamMin=[]  DParamMax=[]  NParamMin=[]  NParamMax=[]  KbParamMin=[]  KbParamMax=[]  KtParamMin=[]  KtParamMax=[]  KbOutMin=[]  KbOutMax=[]  KtOutMin=[]  KtOutMax=[]  IntegratorOutMin=[]  IntegratorOutMax=[]  FilterOutMin=[]  FilterOutMax=[]  SumI1OutMin=[]  SumI1OutMax=[]  SumI2OutMin=[]  SumI2OutMax=[]  SumI3OutMin=[]  SumI3OutMax=[]  SumI4OutMin=[]  SumI4OutMax=[]  SumDOutMin=[]  SumDOutMax=[]  DifferentiatorOutMin=[]  DifferentiatorOutMax=[]  FilterDiffOutCoefMin=[]  FilterDiffOutCoefMax=[]  ReciprocalOutMin=[]  ReciprocalOutMax=[]  SumDenOutMin=[]  SumDenOutMax=[]  SumNumOutMin=[]  SumNumOutMax=[]  DivideOutMin=[]  DivideOutMax=[]  UdiffTsProdOutMin=[]  UdiffTsProdOutMax=[]  NTsProdOutMin=[]  NTsProdOutMax=[]  UintegralTsProdOutMin=[]  UintegralTsProdOutMax=[]  UngainTsProdOutMin=[]  UngainTsProdOutMax=[]  ClampingZeroOutDataTypeStr=Inherit: Inherit via back propagation  ClampingZeroOutMin=[]  ClampingZeroOutMax=[]  FilterDenConstantOutDataTypeStr=Inherit: Inherit via back propagation  FilterDenConstantOutMin=[]  FilterDenConstantOutMax=[]  PCopyOutDataTypeStr=Inherit: Inherit via back propagation  PCopyOutMin=[]  PCopyOutMax=[]  NCopyOutDataTypeStr=Inherit: Inherit via back propagation  NCopyOutMin=[]  NCopyOutMax=[]  IntegratorContinuousStateAttributes=''  IntegratorStateMustResolveToSignalObject=off  IntegratorRTWStateStorageClass=Auto  FilterContinuousStateAttributes=''  FilterStateMustResolveToSignalObject=off  FilterRTWStateStorageClass=Auto  ParallelPVariant=InternalParameters  IdealPVariant=Disabled  IVariant=InternalParameters  DVariant=Disabled  IntegratorVariant=Continuous  SatVariant=Enabled  AWVariant=ContClampingParallel  PCopyVariant=Disabled  TRVariant=Disabled  FdbkBlocksVariant=Forward  IdealPFdbkVariant=Disabled  SatFdbkVariant=Disabled  DerivativeFilterVariant=Disabled  NVariant=Disabled  NCopyVariant=Disabled_SignalSpec  FilterICVariant=Disabled  IntegratorICVariant=InternalICs  ExternalResetVariant=Disabled  TRSumVariant=Passthrough  SumFdbkVariant=Disabled  SumVariant=Sum_PI  TsampFilterVariant=InternalTs  TsampNgainVariant=Passthrough  TsampIntegralVariant=Disabled_SignalSpec  ExternalSaturationOutDataTypeStr=Inherit: Same as second input  DerivativeSourceVariant=Disabled  PreIntVariant=InternalPreInt
  Sum : Sum  Inputs=|+-
  TorqueCmd : Outport
  wires:
  wCmd/1 -> Sum/1
  Sum/1 -> PI Controller/1  "rad/s"
  w/1 -> Sum/2
  PI Controller/1 -> TorqueCmd/1  "N*m"

== system UAV_Research_Environment/UAV Plant/UAV Physical [Simscape]/Motor ESC 2/Speed PI Control ==
  wCmd : Inport
  w : Inport  Port=2
  PI Controller : slpidlib/PID Controller  Controller=PI  Form=Parallel  TimeDomain=Continuous-time  UseExternalTs=off  SampleTime=-1  IntegratorMethod=Forward Euler  FilterMethod=Forward Euler  ControllerParametersSource=internal  P=P_UAV.drive.speed_pi.Kp  I=P_UAV.drive.speed_pi.Ki  UseKiTs=off  D=0.000001  UseExternalDerivativeSource=off  N=10000  UseFilter=on  TunerSelectOption=Transfer Function Based (PID Tuner App)  InitialConditionSource=internal  InitialConditionForIntegrator=0  InitialConditionForFilter=0  DifferentiatorICPrevScaledInput=0  ExternalReset=none  TrackingMode=off  Kt=1  LimitOutput=on  SatLimitsSource=internal  UpperSaturationLimit=P_UAV.drive.speed_pi.torque_limit_Nm  LowerSaturationLimit=-P_UAV.drive.speed_pi.torque_limit_Nm  LinearizeAsGain=on  AntiWindupMode=clamping  Kb=1  LimitIntegrator=off  UpperIntegratorSaturationLimit=inf  LowerIntegratorSaturationLimit=-inf  POutMin=[]  POutMax=[]  IOutMin=[]  IOutMax=[]  DOutMin=[]  DOutMax=[]  NOutMin=[]  NOutMax=[]  SumOutMin=[]  SumOutMax=[]  SaturationOutMin=[]  SaturationOutMax=[]  PParamMin=[]  PParamMax=[]  IParamMin=[]  IParamMax=[]  DParamMin=[]  DParamMax=[]  NParamMin=[]  NParamMax=[]  KbParamMin=[]  KbParamMax=[]  KtParamMin=[]  KtParamMax=[]  KbOutMin=[]  KbOutMax=[]  KtOutMin=[]  KtOutMax=[]  IntegratorOutMin=[]  IntegratorOutMax=[]  FilterOutMin=[]  FilterOutMax=[]  SumI1OutMin=[]  SumI1OutMax=[]  SumI2OutMin=[]  SumI2OutMax=[]  SumI3OutMin=[]  SumI3OutMax=[]  SumI4OutMin=[]  SumI4OutMax=[]  SumDOutMin=[]  SumDOutMax=[]  DifferentiatorOutMin=[]  DifferentiatorOutMax=[]  FilterDiffOutCoefMin=[]  FilterDiffOutCoefMax=[]  ReciprocalOutMin=[]  ReciprocalOutMax=[]  SumDenOutMin=[]  SumDenOutMax=[]  SumNumOutMin=[]  SumNumOutMax=[]  DivideOutMin=[]  DivideOutMax=[]  UdiffTsProdOutMin=[]  UdiffTsProdOutMax=[]  NTsProdOutMin=[]  NTsProdOutMax=[]  UintegralTsProdOutMin=[]  UintegralTsProdOutMax=[]  UngainTsProdOutMin=[]  UngainTsProdOutMax=[]  ClampingZeroOutDataTypeStr=Inherit: Inherit via back propagation  ClampingZeroOutMin=[]  ClampingZeroOutMax=[]  FilterDenConstantOutDataTypeStr=Inherit: Inherit via back propagation  FilterDenConstantOutMin=[]  FilterDenConstantOutMax=[]  PCopyOutDataTypeStr=Inherit: Inherit via back propagation  PCopyOutMin=[]  PCopyOutMax=[]  NCopyOutDataTypeStr=Inherit: Inherit via back propagation  NCopyOutMin=[]  NCopyOutMax=[]  IntegratorContinuousStateAttributes=''  IntegratorStateMustResolveToSignalObject=off  IntegratorRTWStateStorageClass=Auto  FilterContinuousStateAttributes=''  FilterStateMustResolveToSignalObject=off  FilterRTWStateStorageClass=Auto  ParallelPVariant=InternalParameters  IdealPVariant=Disabled  IVariant=InternalParameters  DVariant=Disabled  IntegratorVariant=Continuous  SatVariant=Enabled  AWVariant=ContClampingParallel  PCopyVariant=Disabled  TRVariant=Disabled  FdbkBlocksVariant=Forward  IdealPFdbkVariant=Disabled  SatFdbkVariant=Disabled  DerivativeFilterVariant=Disabled  NVariant=Disabled  NCopyVariant=Disabled_SignalSpec  FilterICVariant=Disabled  IntegratorICVariant=InternalICs  ExternalResetVariant=Disabled  TRSumVariant=Passthrough  SumFdbkVariant=Disabled  SumVariant=Sum_PI  TsampFilterVariant=InternalTs  TsampNgainVariant=Passthrough  TsampIntegralVariant=Disabled_SignalSpec  ExternalSaturationOutDataTypeStr=Inherit: Same as second input  DerivativeSourceVariant=Disabled  PreIntVariant=InternalPreInt
  Sum : Sum  Inputs=|+-
  TorqueCmd : Outport
  wires:
  wCmd/1 -> Sum/1
  Sum/1 -> PI Controller/1  "rad/s"
  w/1 -> Sum/2
  PI Controller/1 -> TorqueCmd/1  "N*m"
